simulink model "model_cnn"  (R2020a)
settings: Solver=VariableStepAuto  StartTime=0.0  StopTime=1e6/fs  RelTol=1e-3
PreLoadFcn:
  | setup_imports;
  | %dense2_numerictype = fixdt(1,18,10);
  | %conv1_numerictype = fixdt(1,18,21);
InitFcn:
  | % Intermediate signal dimensions
  | input_dim = [1, 2, 128];
  | layer1_dim = hInterConvLayerDims([1,3,1,64],input_dim,1); % dims : [C,H,W]
  | layer2_dim = hInterConvLayerDims([2,3,64,16],layer1_dim,1);% dims : [C,H,W]
  | layer3_dim = [1,128];
  | 
  | % Conv Layer 1 dimensions
  | conv1_dims = struct(...
  |     'input_dim',    input_dim,...       input_dim = C,H,W
  |     'filter_dim',   [1, 3, 1, 64],...  filter_dim = K,J,C,N
  |     'stride',       1,...
  |     'row_output',   3,...
  |     'output_dim',   layer1_dim);
  | 
  | % Conv Layer 2 dimensions
  | conv2_dims = struct(...
  |     'input_dim',    layer1_dim,...      input = C,H.W
  |     'filter_dim',   [2, 3, 64, 16],...  filter_dim = K,J,C,N
  |     'stride',       1,...
  |     'row_output',   2*3*64,...
  |     'output_dim',   layer2_dim);
  | 
  | % Dense Layer 1 dimensions
  | dense1_dims = struct(...
  |     'input_dim',    layer2_dim,...      input = C,H,W
  |     'weight_dim',   [1984, 128],...     weight_dim = H,W
  |     'output_dim',   layer3_dim);
  | 
  | % Load saved weights and input
  | setup_imports;
  | 
  | fs = 128e6;
  | fs_axi = 100e6;
  | R = 32;
values from neighbouring files (symbols this model uses):
  datatypeInput = X_test.numerictype    [setup_imports.m]
  gemm_wconv1 = fi(hInterleaveFilters(Wconv1),1,16)    [setup_imports.m]
  gemm_wconv2 = fi(hInterleaveFilters(Wconv2),1,16)    [setup_imports.m]
  wdense1 = fi(Wdense1,1,16)    [setup_imports.m]
  wdense2 = fi(Wdense2,1,16)    [setup_imports.m]
undefined symbols (not defined in the file or in its folder): ltehdlRAMinitPO2
libraries: hdlsllib x1022, dspsigops x3, dspsrcs4 x2
(part 9 of 23)

== system model_cnn/HDL CNN Model/Dense Layer 1/Dense Layer 1/Weight Storage79 ==
  count_Weights : Inport
  Constant : Constant  Value=0  OutDataTypeStr=wdense1.numerictype  SampleTime=-1
  Constant1 : Constant  Value=false  SampleTime=-1
  Single Port RAM System : hdlsllib/HDL RAMs/Single Port RAM System  RAMType=Single port  WriteOutputValue=New data  RAMInitialValue=ltehdlRAMinitPO2(wdense1(:,dim).',2048)  SimulateUsing=Code generation
      settings: SourceProductBaseCode=SL
  Out1 : Outport
  wires:
  Single Port RAM System/1 -> Out1/1
  Constant/1 -> Single Port RAM System/1
  Constant1/1 -> Single Port RAM System/3
  count_Weights/1 -> Single Port RAM System/2

== system model_cnn/HDL CNN Model/Dense Layer 1/Dense Layer 1/Weight Storage8 ==
  count_Weights : Inport
  Constant : Constant  Value=0  OutDataTypeStr=wdense1.numerictype  SampleTime=-1
  Constant1 : Constant  Value=false  SampleTime=-1
  Single Port RAM System : hdlsllib/HDL RAMs/Single Port RAM System  RAMType=Single port  WriteOutputValue=New data  RAMInitialValue=ltehdlRAMinitPO2(wdense1(:,dim).',2048)  SimulateUsing=Code generation
      settings: SourceProductBaseCode=SL
  Out1 : Outport
  wires:
  Single Port RAM System/1 -> Out1/1
  Constant/1 -> Single Port RAM System/1
  Constant1/1 -> Single Port RAM System/3
  count_Weights/1 -> Single Port RAM System/2

== system model_cnn/HDL CNN Model/Dense Layer 1/Dense Layer 1/Weight Storage80 ==
  count_Weights : Inport
  Constant : Constant  Value=0  OutDataTypeStr=wdense1.numerictype  SampleTime=-1
  Constant1 : Constant  Value=false  SampleTime=-1
  Single Port RAM System : hdlsllib/HDL RAMs/Single Port RAM System  RAMType=Single port  WriteOutputValue=New data  RAMInitialValue=ltehdlRAMinitPO2(wdense1(:,dim).',2048)  SimulateUsing=Code generation
      settings: SourceProductBaseCode=SL
  Out1 : Outport
  wires:
  Single Port RAM System/1 -> Out1/1
  Constant/1 -> Single Port RAM System/1
  Constant1/1 -> Single Port RAM System/3
  count_Weights/1 -> Single Port RAM System/2

== system model_cnn/HDL CNN Model/Dense Layer 1/Dense Layer 1/Weight Storage81 ==
  count_Weights : Inport
  Constant : Constant  Value=0  OutDataTypeStr=wdense1.numerictype  SampleTime=-1
  Constant1 : Constant  Value=false  SampleTime=-1
  Single Port RAM System : hdlsllib/HDL RAMs/Single Port RAM System  RAMType=Single port  WriteOutputValue=New data  RAMInitialValue=ltehdlRAMinitPO2(wdense1(:,dim).',2048)  SimulateUsing=Code generation
      settings: SourceProductBaseCode=SL
  Out1 : Outport
  wires:
  Single Port RAM System/1 -> Out1/1
  Constant/1 -> Single Port RAM System/1
  Constant1/1 -> Single Port RAM System/3
  count_Weights/1 -> Single Port RAM System/2

== system model_cnn/HDL CNN Model/Dense Layer 1/Dense Layer 1/Weight Storage82 ==
  count_Weights : Inport
  Constant : Constant  Value=0  OutDataTypeStr=wdense1.numerictype  SampleTime=-1
  Constant1 : Constant  Value=false  SampleTime=-1
  Single Port RAM System : hdlsllib/HDL RAMs/Single Port RAM System  RAMType=Single port  WriteOutputValue=New data  RAMInitialValue=ltehdlRAMinitPO2(wdense1(:,dim).',2048)  SimulateUsing=Code generation
      settings: SourceProductBaseCode=SL
  Out1 : Outport
  wires:
  Single Port RAM System/1 -> Out1/1
  Constant/1 -> Single Port RAM System/1
  Constant1/1 -> Single Port RAM System/3
  count_Weights/1 -> Single Port RAM System/2

== system model_cnn/HDL CNN Model/Dense Layer 1/Dense Layer 1/Weight Storage83 ==
  count_Weights : Inport
  Constant : Constant  Value=0  OutDataTypeStr=wdense1.numerictype  SampleTime=-1
  Constant1 : Constant  Value=false  SampleTime=-1
  Single Port RAM System : hdlsllib/HDL RAMs/Single Port RAM System  RAMType=Single port  WriteOutputValue=New data  RAMInitialValue=ltehdlRAMinitPO2(wdense1(:,dim).',2048)  SimulateUsing=Code generation
      settings: SourceProductBaseCode=SL
  Out1 : Outport
  wires:
  Single Port RAM System/1 -> Out1/1
  Constant/1 -> Single Port RAM System/1
  Constant1/1 -> Single Port RAM System/3
  count_Weights/1 -> Single Port RAM System/2

== system model_cnn/HDL CNN Model/Dense Layer 1/Dense Layer 1/Weight Storage84 ==
  count_Weights : Inport
  Constant : Constant  Value=0  OutDataTypeStr=wdense1.numerictype  SampleTime=-1
  Constant1 : Constant  Value=false  SampleTime=-1
  Single Port RAM System : hdlsllib/HDL RAMs/Single Port RAM System  RAMType=Single port  WriteOutputValue=New data  RAMInitialValue=ltehdlRAMinitPO2(wdense1(:,dim).',2048)  SimulateUsing=Code generation
      settings: SourceProductBaseCode=SL
  Out1 : Outport
  wires:
  Single Port RAM System/1 -> Out1/1
  Constant/1 -> Single Port RAM System/1
  Constant1/1 -> Single Port RAM System/3
  count_Weights/1 -> Single Port RAM System/2

== system model_cnn/HDL CNN Model/Dense Layer 1/Dense Layer 1/Weight Storage85 ==
  count_Weights : Inport
  Constant : Constant  Value=0  OutDataTypeStr=wdense1.numerictype  SampleTime=-1
  Constant1 : Constant  Value=false  SampleTime=-1
  Single Port RAM System : hdlsllib/HDL RAMs/Single Port RAM System  RAMType=Single port  WriteOutputValue=New data  RAMInitialValue=ltehdlRAMinitPO2(wdense1(:,dim).',2048)  SimulateUsing=Code generation
      settings: SourceProductBaseCode=SL
  Out1 : Outport
  wires:
  Single Port RAM System/1 -> Out1/1
  Constant/1 -> Single Port RAM System/1
  Constant1/1 -> Single Port RAM System/3
  count_Weights/1 -> Single Port RAM System/2

== system model_cnn/HDL CNN Model/Dense Layer 1/Dense Layer 1/Weight Storage86 ==
  count_Weights : Inport
  Constant : Constant  Value=0  OutDataTypeStr=wdense1.numerictype  SampleTime=-1
  Constant1 : Constant  Value=false  SampleTime=-1
  Single Port RAM System : hdlsllib/HDL RAMs/Single Port RAM System  RAMType=Single port  WriteOutputValue=New data  RAMInitialValue=ltehdlRAMinitPO2(wdense1(:,dim).',2048)  SimulateUsing=Code generation
      settings: SourceProductBaseCode=SL
  Out1 : Outport
  wires:
  Single Port RAM System/1 -> Out1/1
  Constant/1 -> Single Port RAM System/1
  Constant1/1 -> Single Port RAM System/3
  count_Weights/1 -> Single Port RAM System/2

== system model_cnn/HDL CNN Model/Dense Layer 1/Dense Layer 1/Weight Storage87 ==
  count_Weights : Inport
  Constant : Constant  Value=0  OutDataTypeStr=wdense1.numerictype  SampleTime=-1
  Constant1 : Constant  Value=false  SampleTime=-1
  Single Port RAM System : hdlsllib/HDL RAMs/Single Port RAM System  RAMType=Single port  WriteOutputValue=New data  RAMInitialValue=ltehdlRAMinitPO2(wdense1(:,dim).',2048)  SimulateUsing=Code generation
      settings: SourceProductBaseCode=SL
  Out1 : Outport
  wires:
  Single Port RAM System/1 -> Out1/1
  Constant/1 -> Single Port RAM System/1
  Constant1/1 -> Single Port RAM System/3
  count_Weights/1 -> Single Port RAM System/2

== system model_cnn/HDL CNN Model/Dense Layer 1/Dense Layer 1/Weight Storage88 ==
  count_Weights : Inport
  Constant : Constant  Value=0  OutDataTypeStr=wdense1.numerictype  SampleTime=-1
  Constant1 : Constant  Value=false  SampleTime=-1
  Single Port RAM System : hdlsllib/HDL RAMs/Single Port RAM System  RAMType=Single port  WriteOutputValue=New data  RAMInitialValue=ltehdlRAMinitPO2(wdense1(:,dim).',2048)  SimulateUsing=Code generation
      settings: SourceProductBaseCode=SL
  Out1 : Outport
  wires:
  Single Port RAM System/1 -> Out1/1
  Constant/1 -> Single Port RAM System/1
  Constant1/1 -> Single Port RAM System/3
  count_Weights/1 -> Single Port RAM System/2

== system model_cnn/HDL CNN Model/Dense Layer 1/Dense Layer 1/Weight Storage89 ==
  count_Weights : Inport
  Constant : Constant  Value=0  OutDataTypeStr=wdense1.numerictype  SampleTime=-1
  Constant1 : Constant  Value=false  SampleTime=-1
  Single Port RAM System : hdlsllib/HDL RAMs/Single Port RAM System  RAMType=Single port  WriteOutputValue=New data  RAMInitialValue=ltehdlRAMinitPO2(wdense1(:,dim).',2048)  SimulateUsing=Code generation
      settings: SourceProductBaseCode=SL
  Out1 : Outport
  wires:
  Single Port RAM System/1 -> Out1/1
  Constant/1 -> Single Port RAM System/1
  Constant1/1 -> Single Port RAM System/3
  count_Weights/1 -> Single Port RAM System/2

== system model_cnn/HDL CNN Model/Dense Layer 1/Dense Layer 1/Weight Storage9 ==
  count_Weights : Inport
  Constant : Constant  Value=0  OutDataTypeStr=wdense1.numerictype  SampleTime=-1
  Constant1 : Constant  Value=false  SampleTime=-1
  Single Port RAM System : hdlsllib/HDL RAMs/Single Port RAM System  RAMType=Single port  WriteOutputValue=New data  RAMInitialValue=ltehdlRAMinitPO2(wdense1(:,dim).',2048)  SimulateUsing=Code generation
      settings: SourceProductBaseCode=SL
  Out1 : Outport
  wires:
  Single Port RAM System/1 -> Out1/1
  Constant/1 -> Single Port RAM System/1
  Constant1/1 -> Single Port RAM System/3
  count_Weights/1 -> Single Port RAM System/2

== system model_cnn/HDL CNN Model/Dense Layer 1/Dense Layer 1/Weight Storage90 ==
  count_Weights : Inport
  Constant : Constant  Value=0  OutDataTypeStr=wdense1.numerictype  SampleTime=-1
  Constant1 : Constant  Value=false  SampleTime=-1
  Single Port RAM System : hdlsllib/HDL RAMs/Single Port RAM System  RAMType=Single port  WriteOutputValue=New data  RAMInitialValue=ltehdlRAMinitPO2(wdense1(:,dim).',2048)  SimulateUsing=Code generation
      settings: SourceProductBaseCode=SL
  Out1 : Outport
  wires:
  Single Port RAM System/1 -> Out1/1
  Constant/1 -> Single Port RAM System/1
  Constant1/1 -> Single Port RAM System/3
  count_Weights/1 -> Single Port RAM System/2

== system model_cnn/HDL CNN Model/Dense Layer 1/Dense Layer 1/Weight Storage91 ==
  count_Weights : Inport
  Constant : Constant  Value=0  OutDataTypeStr=wdense1.numerictype  SampleTime=-1
  Constant1 : Constant  Value=false  SampleTime=-1
  Single Port RAM System : hdlsllib/HDL RAMs/Single Port RAM System  RAMType=Single port  WriteOutputValue=New data  RAMInitialValue=ltehdlRAMinitPO2(wdense1(:,dim).',2048)  SimulateUsing=Code generation
      settings: SourceProductBaseCode=SL
  Out1 : Outport
  wires:
  Single Port RAM System/1 -> Out1/1
  Constant/1 -> Single Port RAM System/1
  Constant1/1 -> Single Port RAM System/3
  count_Weights/1 -> Single Port RAM System/2

== system model_cnn/HDL CNN Model/Dense Layer 1/Dense Layer 1/Weight Storage92 ==
  count_Weights : Inport
  Constant : Constant  Value=0  OutDataTypeStr=wdense1.numerictype  SampleTime=-1
  Constant1 : Constant  Value=false  SampleTime=-1
  Single Port RAM System : hdlsllib/HDL RAMs/Single Port RAM System  RAMType=Single port  WriteOutputValue=New data  RAMInitialValue=ltehdlRAMinitPO2(wdense1(:,dim).',2048)  SimulateUsing=Code generation
      settings: SourceProductBaseCode=SL
  Out1 : Outport
  wires:
  Single Port RAM System/1 -> Out1/1
  Constant/1 -> Single Port RAM System/1
  Constant1/1 -> Single Port RAM System/3
  count_Weights/1 -> Single Port RAM System/2

== system model_cnn/HDL CNN Model/Dense Layer 1/Dense Layer 1/Weight Storage93 ==
  count_Weights : Inport
  Constant : Constant  Value=0  OutDataTypeStr=wdense1.numerictype  SampleTime=-1
  Constant1 : Constant  Value=false  SampleTime=-1
  Single Port RAM System : hdlsllib/HDL RAMs/Single Port RAM System  RAMType=Single port  WriteOutputValue=New data  RAMInitialValue=ltehdlRAMinitPO2(wdense1(:,dim).',2048)  SimulateUsing=Code generation
      settings: SourceProductBaseCode=SL
  Out1 : Outport
  wires:
  Single Port RAM System/1 -> Out1/1
  Constant/1 -> Single Port RAM System/1
  Constant1/1 -> Single Port RAM System/3
  count_Weights/1 -> Single Port RAM System/2

== system model_cnn/HDL CNN Model/Dense Layer 1/Dense Layer 1/Weight Storage94 ==
  count_Weights : Inport
  Constant : Constant  Value=0  OutDataTypeStr=wdense1.numerictype  SampleTime=-1
  Constant1 : Constant  Value=false  SampleTime=-1
  Single Port RAM System : hdlsllib/HDL RAMs/Single Port RAM System  RAMType=Single port  WriteOutputValue=New data  RAMInitialValue=ltehdlRAMinitPO2(wdense1(:,dim).',2048)  SimulateUsing=Code generation
      settings: SourceProductBaseCode=SL
  Out1 : Outport
  wires:
  Single Port RAM System/1 -> Out1/1
  Constant/1 -> Single Port RAM System/1
  Constant1/1 -> Single Port RAM System/3
  count_Weights/1 -> Single Port RAM System/2

== system model_cnn/HDL CNN Model/Dense Layer 1/Dense Layer 1/Weight Storage95 ==
  count_Weights : Inport
  Constant : Constant  Value=0  OutDataTypeStr=wdense1.numerictype  SampleTime=-1
  Constant1 : Constant  Value=false  SampleTime=-1
  Single Port RAM System : hdlsllib/HDL RAMs/Single Port RAM System  RAMType=Single port  WriteOutputValue=New data  RAMInitialValue=ltehdlRAMinitPO2(wdense1(:,dim).',2048)  SimulateUsing=Code generation
      settings: SourceProductBaseCode=SL
  Out1 : Outport
  wires:
  Single Port RAM System/1 -> Out1/1
  Constant/1 -> Single Port RAM System/1
  Constant1/1 -> Single Port RAM System/3
  count_Weights/1 -> Single Port RAM System/2

== system model_cnn/HDL CNN Model/Dense Layer 1/Dense Layer 1/Weight Storage96 ==
  count_Weights : Inport
  Constant : Constant  Value=0  OutDataTypeStr=wdense1.numerictype  SampleTime=-1
  Constant1 : Constant  Value=false  SampleTime=-1
  Single Port RAM System : hdlsllib/HDL RAMs/Single Port RAM System  RAMType=Single port  WriteOutputValue=New data  RAMInitialValue=ltehdlRAMinitPO2(wdense1(:,dim).',2048)  SimulateUsing=Code generation
      settings: SourceProductBaseCode=SL
  Out1 : Outport
  wires:
  Single Port RAM System/1 -> Out1/1
  Constant/1 -> Single Port RAM System/1
  Constant1/1 -> Single Port RAM System/3
  count_Weights/1 -> Single Port RAM System/2

== system model_cnn/HDL CNN Model/Dense Layer 1/Dense Layer 1/Weight Storage97 ==
  count_Weights : Inport
  Constant : Constant  Value=0  OutDataTypeStr=wdense1.numerictype  SampleTime=-1
  Constant1 : Constant  Value=false  SampleTime=-1
  Single Port RAM System : hdlsllib/HDL RAMs/Single Port RAM System  RAMType=Single port  WriteOutputValue=New data  RAMInitialValue=ltehdlRAMinitPO2(wdense1(:,dim).',2048)  SimulateUsing=Code generation
      settings: SourceProductBaseCode=SL
  Out1 : Outport
  wires:
  Single Port RAM System/1 -> Out1/1
  Constant/1 -> Single Port RAM System/1
  Constant1/1 -> Single Port RAM System/3
  count_Weights/1 -> Single Port RAM System/2

== system model_cnn/HDL CNN Model/Dense Layer 1/Dense Layer 1/Weight Storage98 ==
  count_Weights : Inport
  Constant : Constant  Value=0  OutDataTypeStr=wdense1.numerictype  SampleTime=-1
  Constant1 : Constant  Value=false  SampleTime=-1
  Single Port RAM System : hdlsllib/HDL RAMs/Single Port RAM System  RAMType=Single port  WriteOutputValue=New data  RAMInitialValue=ltehdlRAMinitPO2(wdense1(:,dim).',2048)  SimulateUsing=Code generation
      settings: SourceProductBaseCode=SL
  Out1 : Outport
  wires:
  Single Port RAM System/1 -> Out1/1
  Constant/1 -> Single Port RAM System/1
  Constant1/1 -> Single Port RAM System/3
  count_Weights/1 -> Single Port RAM System/2

== system model_cnn/HDL CNN Model/Dense Layer 1/Dense Layer 1/Weight Storage99 ==
  count_Weights : Inport
  Constant : Constant  Value=0  OutDataTypeStr=wdense1.numerictype  SampleTime=-1
  Constant1 : Constant  Value=false  SampleTime=-1
  Single Port RAM System : hdlsllib/HDL RAMs/Single Port RAM System  RAMType=Single port  WriteOutputValue=New data  RAMInitialValue=ltehdlRAMinitPO2(wdense1(:,dim).',2048)  SimulateUsing=Code generation
      settings: SourceProductBaseCode=SL
  Out1 : Outport
  wires:
  Single Port RAM System/1 -> Out1/1
  Constant/1 -> Single Port RAM System/1
  Constant1/1 -> Single Port RAM System/3
  count_Weights/1 -> Single Port RAM System/2

== system model_cnn/HDL CNN Model/Dense Layer 1/Dense Layer 1/adder 0 ==
  In1 : Inport
  In2 : Inport  Port=2
  In3 : Inport  Port=3
  Data Type Conversion : DataTypeConversion  OutDataTypeStr=datatypeLayer3
  Multiply-Accumulate : hdlsllib/HDL Operations/Multiply-Accumulate  opMode=Streaming - using Number of Samples  initValueSetting=Dialog  initValue=0  initValueSetting2=Dialog  initValue2=0  initValueSetting3=Dialog  initValue3=0  num_samples=1984  RndMeth2=Floor  RndMeth3=Floor  datatype2=Inherit: Inherit via back propagation  datatype3=accumoutdatatype3  validOut=on  endInandOut=on  startOut=on  countOut=on  dim=-1  DoSatur=off  parallel=off
      settings: SourceProductBaseCode=SL
  Terminator : Terminator
  Terminator1 : Terminator
  dataOut : Outport
  validOut : Outport  Port=2
  wires:
  ? -> validOut/1  "vectorOutValid"
  In1/1 -> Multiply-Accumulate/2
  ? -> Terminator/1  "countOut"
  Multiply-Accumulate/1 -> Data Type Conversion/1
  In3/1 -> ?
  In2/1 -> Multiply-Accumulate/1
  ? -> Terminator1/1  "validOut"
  Data Type Conversion/1 -> dataOut/1

== system model_cnn/HDL CNN Model/Dense Layer 1/Dense Layer 1/adder1 ==
  In1 : Inport
  In2 : Inport  Port=2
  In3 : Inport  Port=3
  Data Type Conversion : DataTypeConversion  OutDataTypeStr=datatypeLayer3
  Multiply-Accumulate : hdlsllib/HDL Operations/Multiply-Accumulate  opMode=Streaming - using Number of Samples  initValueSetting=Dialog  initValue=0  initValueSetting2=Dialog  initValue2=0  initValueSetting3=Dialog  initValue3=0  num_samples=1984  RndMeth2=Floor  RndMeth3=Floor  datatype2=Inherit: Inherit via back propagation  datatype3=accumoutdatatype3  validOut=on  endInandOut=on  startOut=on  countOut=on  dim=-1  DoSatur=off  parallel=off
      settings: SourceProductBaseCode=SL
  Terminator : Terminator
  Terminator1 : Terminator
  Terminator2 : Terminator
  dataOut : Outport
  wires:
  Data Type Conversion/1 -> dataOut/1
  ? -> Terminator1/1  "validOut"
  In2/1 -> Multiply-Accumulate/1
  In3/1 -> ?
  Multiply-Accumulate/1 -> Data Type Conversion/1
  ? -> Terminator/1  "countOut"
  In1/1 -> Multiply-Accumulate/2
  ? -> Terminator2/1  "vectorOutValid"

== system model_cnn/HDL CNN Model/Dense Layer 1/Dense Layer 1/adder10 ==
  In1 : Inport
  In2 : Inport  Port=2
  In3 : Inport  Port=3
  Data Type Conversion : DataTypeConversion  OutDataTypeStr=datatypeLayer3
  Multiply-Accumulate : hdlsllib/HDL Operations/Multiply-Accumulate  opMode=Streaming - using Number of Samples  initValueSetting=Dialog  initValue=0  initValueSetting2=Dialog  initValue2=0  initValueSetting3=Dialog  initValue3=0  num_samples=1984  RndMeth2=Floor  RndMeth3=Floor  datatype2=Inherit: Inherit via back propagation  datatype3=accumoutdatatype3  validOut=on  endInandOut=on  startOut=on  countOut=on  dim=-1  DoSatur=off  parallel=off
      settings: SourceProductBaseCode=SL
  Terminator : Terminator
  Terminator1 : Terminator
  Terminator2 : Terminator
  dataOut : Outport
  wires:
  Data Type Conversion/1 -> dataOut/1
  ? -> Terminator1/1  "validOut"
  In2/1 -> Multiply-Accumulate/1
  In3/1 -> ?
  Multiply-Accumulate/1 -> Data Type Conversion/1
  ? -> Terminator/1  "countOut"
  In1/1 -> Multiply-Accumulate/2
  ? -> Terminator2/1  "vectorOutValid"

== system model_cnn/HDL CNN Model/Dense Layer 1/Dense Layer 1/adder100 ==
  In1 : Inport
  In2 : Inport  Port=2
  In3 : Inport  Port=3
  Data Type Conversion : DataTypeConversion  OutDataTypeStr=datatypeLayer3
  Multiply-Accumulate : hdlsllib/HDL Operations/Multiply-Accumulate  opMode=Streaming - using Number of Samples  initValueSetting=Dialog  initValue=0  initValueSetting2=Dialog  initValue2=0  initValueSetting3=Dialog  initValue3=0  num_samples=1984  RndMeth2=Floor  RndMeth3=Floor  datatype2=Inherit: Inherit via back propagation  datatype3=accumoutdatatype3  validOut=on  endInandOut=on  startOut=on  countOut=on  dim=-1  DoSatur=off  parallel=off
      settings: SourceProductBaseCode=SL
  Terminator : Terminator
  Terminator1 : Terminator
  Terminator2 : Terminator
  dataOut : Outport
  wires:
  Data Type Conversion/1 -> dataOut/1
  ? -> Terminator1/1  "validOut"
  In2/1 -> Multiply-Accumulate/1
  In3/1 -> ?
  Multiply-Accumulate/1 -> Data Type Conversion/1
  ? -> Terminator/1  "countOut"
  In1/1 -> Multiply-Accumulate/2
  ? -> Terminator2/1  "vectorOutValid"

== system model_cnn/HDL CNN Model/Dense Layer 1/Dense Layer 1/adder101 ==
  In1 : Inport
  In2 : Inport  Port=2
  In3 : Inport  Port=3
  Data Type Conversion : DataTypeConversion  OutDataTypeStr=datatypeLayer3
  Multiply-Accumulate : hdlsllib/HDL Operations/Multiply-Accumulate  opMode=Streaming - using Number of Samples  initValueSetting=Dialog  initValue=0  initValueSetting2=Dialog  initValue2=0  initValueSetting3=Dialog  initValue3=0  num_samples=1984  RndMeth2=Floor  RndMeth3=Floor  datatype2=Inherit: Inherit via back propagation  datatype3=accumoutdatatype3  validOut=on  endInandOut=on  startOut=on  countOut=on  dim=-1  DoSatur=off  parallel=off
      settings: SourceProductBaseCode=SL
  Terminator : Terminator
  Terminator1 : Terminator
  Terminator2 : Terminator
  dataOut : Outport
  wires:
  Data Type Conversion/1 -> dataOut/1
  ? -> Terminator1/1  "validOut"
  In2/1 -> Multiply-Accumulate/1
  In3/1 -> ?
  Multiply-Accumulate/1 -> Data Type Conversion/1
  ? -> Terminator/1  "countOut"
  In1/1 -> Multiply-Accumulate/2
  ? -> Terminator2/1  "vectorOutValid"

== system model_cnn/HDL CNN Model/Dense Layer 1/Dense Layer 1/adder102 ==
  In1 : Inport
  In2 : Inport  Port=2
  In3 : Inport  Port=3
  Data Type Conversion : DataTypeConversion  OutDataTypeStr=datatypeLayer3
  Multiply-Accumulate : hdlsllib/HDL Operations/Multiply-Accumulate  opMode=Streaming - using Number of Samples  initValueSetting=Dialog  initValue=0  initValueSetting2=Dialog  initValue2=0  initValueSetting3=Dialog  initValue3=0  num_samples=1984  RndMeth2=Floor  RndMeth3=Floor  datatype2=Inherit: Inherit via back propagation  datatype3=accumoutdatatype3  validOut=on  endInandOut=on  startOut=on  countOut=on  dim=-1  DoSatur=off  parallel=off
      settings: SourceProductBaseCode=SL
  Terminator : Terminator
  Terminator1 : Terminator
  Terminator2 : Terminator
  dataOut : Outport
  wires:
  Data Type Conversion/1 -> dataOut/1
  ? -> Terminator1/1  "validOut"
  In2/1 -> Multiply-Accumulate/1
  In3/1 -> ?
  Multiply-Accumulate/1 -> Data Type Conversion/1
  ? -> Terminator/1  "countOut"
  In1/1 -> Multiply-Accumulate/2
  ? -> Terminator2/1  "vectorOutValid"

== system model_cnn/HDL CNN Model/Dense Layer 1/Dense Layer 1/adder103 ==
  In1 : Inport
  In2 : Inport  Port=2
  In3 : Inport  Port=3
  Data Type Conversion : DataTypeConversion  OutDataTypeStr=datatypeLayer3
  Multiply-Accumulate : hdlsllib/HDL Operations/Multiply-Accumulate  opMode=Streaming - using Number of Samples  initValueSetting=Dialog  initValue=0  initValueSetting2=Dialog  initValue2=0  initValueSetting3=Dialog  initValue3=0  num_samples=1984  RndMeth2=Floor  RndMeth3=Floor  datatype2=Inherit: Inherit via back propagation  datatype3=accumoutdatatype3  validOut=on  endInandOut=on  startOut=on  countOut=on  dim=-1  DoSatur=off  parallel=off
      settings: SourceProductBaseCode=SL
  Terminator : Terminator
  Terminator1 : Terminator
  Terminator2 : Terminator
  dataOut : Outport
  wires:
  Data Type Conversion/1 -> dataOut/1
  ? -> Terminator1/1  "validOut"
  In2/1 -> Multiply-Accumulate/1
  In3/1 -> ?
  Multiply-Accumulate/1 -> Data Type Conversion/1
  ? -> Terminator/1  "countOut"
  In1/1 -> Multiply-Accumulate/2
  ? -> Terminator2/1  "vectorOutValid"

== system model_cnn/HDL CNN Model/Dense Layer 1/Dense Layer 1/adder104 ==
  In1 : Inport
  In2 : Inport  Port=2
  In3 : Inport  Port=3
  Data Type Conversion : DataTypeConversion  OutDataTypeStr=datatypeLayer3
  Multiply-Accumulate : hdlsllib/HDL Operations/Multiply-Accumulate  opMode=Streaming - using Number of Samples  initValueSetting=Dialog  initValue=0  initValueSetting2=Dialog  initValue2=0  initValueSetting3=Dialog  initValue3=0  num_samples=1984  RndMeth2=Floor  RndMeth3=Floor  datatype2=Inherit: Inherit via back propagation  datatype3=accumoutdatatype3  validOut=on  endInandOut=on  startOut=on  countOut=on  dim=-1  DoSatur=off  parallel=off
      settings: SourceProductBaseCode=SL
  Terminator : Terminator
  Terminator1 : Terminator
  Terminator2 : Terminator
  dataOut : Outport
  wires:
  Data Type Conversion/1 -> dataOut/1
  ? -> Terminator1/1  "validOut"
  In2/1 -> Multiply-Accumulate/1
  In3/1 -> ?
  Multiply-Accumulate/1 -> Data Type Conversion/1
  ? -> Terminator/1  "countOut"
  In1/1 -> Multiply-Accumulate/2
  ? -> Terminator2/1  "vectorOutValid"

== system model_cnn/HDL CNN Model/Dense Layer 1/Dense Layer 1/adder105 ==
  In1 : Inport
  In2 : Inport  Port=2
  In3 : Inport  Port=3
  Data Type Conversion : DataTypeConversion  OutDataTypeStr=datatypeLayer3
  Multiply-Accumulate : hdlsllib/HDL Operations/Multiply-Accumulate  opMode=Streaming - using Number of Samples  initValueSetting=Dialog  initValue=0  initValueSetting2=Dialog  initValue2=0  initValueSetting3=Dialog  initValue3=0  num_samples=1984  RndMeth2=Floor  RndMeth3=Floor  datatype2=Inherit: Inherit via back propagation  datatype3=accumoutdatatype3  validOut=on  endInandOut=on  startOut=on  countOut=on  dim=-1  DoSatur=off  parallel=off
      settings: SourceProductBaseCode=SL
  Terminator : Terminator
  Terminator1 : Terminator
  Terminator2 : Terminator
  dataOut : Outport
  wires:
  Data Type Conversion/1 -> dataOut/1
  ? -> Terminator1/1  "validOut"
  In2/1 -> Multiply-Accumulate/1
  In3/1 -> ?
  Multiply-Accumulate/1 -> Data Type Conversion/1
  ? -> Terminator/1  "countOut"
  In1/1 -> Multiply-Accumulate/2
  ? -> Terminator2/1  "vectorOutValid"

== system model_cnn/HDL CNN Model/Dense Layer 1/Dense Layer 1/adder106 ==
  In1 : Inport
  In2 : Inport  Port=2
  In3 : Inport  Port=3
  Data Type Conversion : DataTypeConversion  OutDataTypeStr=datatypeLayer3
  Multiply-Accumulate : hdlsllib/HDL Operations/Multiply-Accumulate  opMode=Streaming - using Number of Samples  initValueSetting=Dialog  initValue=0  initValueSetting2=Dialog  initValue2=0  initValueSetting3=Dialog  initValue3=0  num_samples=1984  RndMeth2=Floor  RndMeth3=Floor  datatype2=Inherit: Inherit via back propagation  datatype3=accumoutdatatype3  validOut=on  endInandOut=on  startOut=on  countOut=on  dim=-1  DoSatur=off  parallel=off
      settings: SourceProductBaseCode=SL
  Terminator : Terminator
  Terminator1 : Terminator
  Terminator2 : Terminator
  dataOut : Outport
  wires:
  Data Type Conversion/1 -> dataOut/1
  ? -> Terminator1/1  "validOut"
  In2/1 -> Multiply-Accumulate/1
  In3/1 -> ?
  Multiply-Accumulate/1 -> Data Type Conversion/1
  ? -> Terminator/1  "countOut"
  In1/1 -> Multiply-Accumulate/2
  ? -> Terminator2/1  "vectorOutValid"

== system model_cnn/HDL CNN Model/Dense Layer 1/Dense Layer 1/adder107 ==
  In1 : Inport
  In2 : Inport  Port=2
  In3 : Inport  Port=3
  Data Type Conversion : DataTypeConversion  OutDataTypeStr=datatypeLayer3
  Multiply-Accumulate : hdlsllib/HDL Operations/Multiply-Accumulate  opMode=Streaming - using Number of Samples  initValueSetting=Dialog  initValue=0  initValueSetting2=Dialog  initValue2=0  initValueSetting3=Dialog  initValue3=0  num_samples=1984  RndMeth2=Floor  RndMeth3=Floor  datatype2=Inherit: Inherit via back propagation  datatype3=accumoutdatatype3  validOut=on  endInandOut=on  startOut=on  countOut=on  dim=-1  DoSatur=off  parallel=off
      settings: SourceProductBaseCode=SL
  Terminator : Terminator
  Terminator1 : Terminator
  Terminator2 : Terminator
  dataOut : Outport
  wires:
  Data Type Conversion/1 -> dataOut/1
  ? -> Terminator1/1  "validOut"
  In2/1 -> Multiply-Accumulate/1
  In3/1 -> ?
  Multiply-Accumulate/1 -> Data Type Conversion/1
  ? -> Terminator/1  "countOut"
  In1/1 -> Multiply-Accumulate/2
  ? -> Terminator2/1  "vectorOutValid"

== system model_cnn/HDL CNN Model/Dense Layer 1/Dense Layer 1/adder108 ==
  In1 : Inport
  In2 : Inport  Port=2
  In3 : Inport  Port=3
  Data Type Conversion : DataTypeConversion  OutDataTypeStr=datatypeLayer3
  Multiply-Accumulate : hdlsllib/HDL Operations/Multiply-Accumulate  opMode=Streaming - using Number of Samples  initValueSetting=Dialog  initValue=0  initValueSetting2=Dialog  initValue2=0  initValueSetting3=Dialog  initValue3=0  num_samples=1984  RndMeth2=Floor  RndMeth3=Floor  datatype2=Inherit: Inherit via back propagation  datatype3=accumoutdatatype3  validOut=on  endInandOut=on  startOut=on  countOut=on  dim=-1  DoSatur=off  parallel=off
      settings: SourceProductBaseCode=SL
  Terminator : Terminator
  Terminator1 : Terminator
  Terminator2 : Terminator
  dataOut : Outport
  wires:
  Data Type Conversion/1 -> dataOut/1
  ? -> Terminator1/1  "validOut"
  In2/1 -> Multiply-Accumulate/1
  In3/1 -> ?
  Multiply-Accumulate/1 -> Data Type Conversion/1
  ? -> Terminator/1  "countOut"
  In1/1 -> Multiply-Accumulate/2
  ? -> Terminator2/1  "vectorOutValid"

== system model_cnn/HDL CNN Model/Dense Layer 1/Dense Layer 1/adder109 ==
  In1 : Inport
  In2 : Inport  Port=2
  In3 : Inport  Port=3
  Data Type Conversion : DataTypeConversion  OutDataTypeStr=datatypeLayer3
  Multiply-Accumulate : hdlsllib/HDL Operations/Multiply-Accumulate  opMode=Streaming - using Number of Samples  initValueSetting=Dialog  initValue=0  initValueSetting2=Dialog  initValue2=0  initValueSetting3=Dialog  initValue3=0  num_samples=1984  RndMeth2=Floor  RndMeth3=Floor  datatype2=Inherit: Inherit via back propagation  datatype3=accumoutdatatype3  validOut=on  endInandOut=on  startOut=on  countOut=on  dim=-1  DoSatur=off  parallel=off
      settings: SourceProductBaseCode=SL
  Terminator : Terminator
  Terminator1 : Terminator
  Terminator2 : Terminator
  dataOut : Outport
  wires:
  Data Type Conversion/1 -> dataOut/1
  ? -> Terminator1/1  "validOut"
  In2/1 -> Multiply-Accumulate/1
  In3/1 -> ?
  Multiply-Accumulate/1 -> Data Type Conversion/1
  ? -> Terminator/1  "countOut"
  In1/1 -> Multiply-Accumulate/2
  ? -> Terminator2/1  "vectorOutValid"

== system model_cnn/HDL CNN Model/Dense Layer 1/Dense Layer 1/adder11 ==
  In1 : Inport
  In2 : Inport  Port=2
  In3 : Inport  Port=3
  Data Type Conversion : DataTypeConversion  OutDataTypeStr=datatypeLayer3
  Multiply-Accumulate : hdlsllib/HDL Operations/Multiply-Accumulate  opMode=Streaming - using Number of Samples  initValueSetting=Dialog  initValue=0  initValueSetting2=Dialog  initValue2=0  initValueSetting3=Dialog  initValue3=0  num_samples=1984  RndMeth2=Floor  RndMeth3=Floor  datatype2=Inherit: Inherit via back propagation  datatype3=accumoutdatatype3  validOut=on  endInandOut=on  startOut=on  countOut=on  dim=-1  DoSatur=off  parallel=off
      settings: SourceProductBaseCode=SL
  Terminator : Terminator
  Terminator1 : Terminator
  Terminator2 : Terminator
  dataOut : Outport
  wires:
  Data Type Conversion/1 -> dataOut/1
  ? -> Terminator1/1  "validOut"
  In2/1 -> Multiply-Accumulate/1
  In3/1 -> ?
  Multiply-Accumulate/1 -> Data Type Conversion/1
  ? -> Terminator/1  "countOut"
  In1/1 -> Multiply-Accumulate/2
  ? -> Terminator2/1  "vectorOutValid"

== system model_cnn/HDL CNN Model/Dense Layer 1/Dense Layer 1/adder110 ==
  In1 : Inport
  In2 : Inport  Port=2
  In3 : Inport  Port=3
  Data Type Conversion : DataTypeConversion  OutDataTypeStr=datatypeLayer3
  Multiply-Accumulate : hdlsllib/HDL Operations/Multiply-Accumulate  opMode=Streaming - using Number of Samples  initValueSetting=Dialog  initValue=0  initValueSetting2=Dialog  initValue2=0  initValueSetting3=Dialog  initValue3=0  num_samples=1984  RndMeth2=Floor  RndMeth3=Floor  datatype2=Inherit: Inherit via back propagation  datatype3=accumoutdatatype3  validOut=on  endInandOut=on  startOut=on  countOut=on  dim=-1  DoSatur=off  parallel=off
      settings: SourceProductBaseCode=SL
  Terminator : Terminator
  Terminator1 : Terminator
  Terminator2 : Terminator
  dataOut : Outport
  wires:
  Data Type Conversion/1 -> dataOut/1
  ? -> Terminator1/1  "validOut"
  In2/1 -> Multiply-Accumulate/1
  In3/1 -> ?
  Multiply-Accumulate/1 -> Data Type Conversion/1
  ? -> Terminator/1  "countOut"
  In1/1 -> Multiply-Accumulate/2
  ? -> Terminator2/1  "vectorOutValid"

== system model_cnn/HDL CNN Model/Dense Layer 1/Dense Layer 1/adder111 ==
  In1 : Inport
  In2 : Inport  Port=2
  In3 : Inport  Port=3
  Data Type Conversion : DataTypeConversion  OutDataTypeStr=datatypeLayer3
  Multiply-Accumulate : hdlsllib/HDL Operations/Multiply-Accumulate  opMode=Streaming - using Number of Samples  initValueSetting=Dialog  initValue=0  initValueSetting2=Dialog  initValue2=0  initValueSetting3=Dialog  initValue3=0  num_samples=1984  RndMeth2=Floor  RndMeth3=Floor  datatype2=Inherit: Inherit via back propagation  datatype3=accumoutdatatype3  validOut=on  endInandOut=on  startOut=on  countOut=on  dim=-1  DoSatur=off  parallel=off
      settings: SourceProductBaseCode=SL
  Terminator : Terminator
  Terminator1 : Terminator
  Terminator2 : Terminator
  dataOut : Outport
  wires:
  Data Type Conversion/1 -> dataOut/1
  ? -> Terminator1/1  "validOut"
  In2/1 -> Multiply-Accumulate/1
  In3/1 -> ?
  Multiply-Accumulate/1 -> Data Type Conversion/1
  ? -> Terminator/1  "countOut"
  In1/1 -> Multiply-Accumulate/2
  ? -> Terminator2/1  "vectorOutValid"

== system model_cnn/HDL CNN Model/Dense Layer 1/Dense Layer 1/adder112 ==
  In1 : Inport
  In2 : Inport  Port=2
  In3 : Inport  Port=3
  Data Type Conversion : DataTypeConversion  OutDataTypeStr=datatypeLayer3
  Multiply-Accumulate : hdlsllib/HDL Operations/Multiply-Accumulate  opMode=Streaming - using Number of Samples  initValueSetting=Dialog  initValue=0  initValueSetting2=Dialog  initValue2=0  initValueSetting3=Dialog  initValue3=0  num_samples=1984  RndMeth2=Floor  RndMeth3=Floor  datatype2=Inherit: Inherit via back propagation  datatype3=accumoutdatatype3  validOut=on  endInandOut=on  startOut=on  countOut=on  dim=-1  DoSatur=off  parallel=off
      settings: SourceProductBaseCode=SL
  Terminator : Terminator
  Terminator1 : Terminator
  Terminator2 : Terminator
  dataOut : Outport
  wires:
  Data Type Conversion/1 -> dataOut/1
  ? -> Terminator1/1  "validOut"
  In2/1 -> Multiply-Accumulate/1
  In3/1 -> ?
  Multiply-Accumulate/1 -> Data Type Conversion/1
  ? -> Terminator/1  "countOut"
  In1/1 -> Multiply-Accumulate/2
  ? -> Terminator2/1  "vectorOutValid"

== system model_cnn/HDL CNN Model/Dense Layer 1/Dense Layer 1/adder113 ==
  In1 : Inport
  In2 : Inport  Port=2
  In3 : Inport  Port=3
  Data Type Conversion : DataTypeConversion  OutDataTypeStr=datatypeLayer3
  Multiply-Accumulate : hdlsllib/HDL Operations/Multiply-Accumulate  opMode=Streaming - using Number of Samples  initValueSetting=Dialog  initValue=0  initValueSetting2=Dialog  initValue2=0  initValueSetting3=Dialog  initValue3=0  num_samples=1984  RndMeth2=Floor  RndMeth3=Floor  datatype2=Inherit: Inherit via back propagation  datatype3=accumoutdatatype3  validOut=on  endInandOut=on  startOut=on  countOut=on  dim=-1  DoSatur=off  parallel=off
      settings: SourceProductBaseCode=SL
  Terminator : Terminator
  Terminator1 : Terminator
  Terminator2 : Terminator
  dataOut : Outport
  wires:
  Data Type Conversion/1 -> dataOut/1
  ? -> Terminator1/1  "validOut"
  In2/1 -> Multiply-Accumulate/1
  In3/1 -> ?
  Multiply-Accumulate/1 -> Data Type Conversion/1
  ? -> Terminator/1  "countOut"
  In1/1 -> Multiply-Accumulate/2
  ? -> Terminator2/1  "vectorOutValid"

== system model_cnn/HDL CNN Model/Dense Layer 1/Dense Layer 1/adder114 ==
  In1 : Inport
  In2 : Inport  Port=2
  In3 : Inport  Port=3
  Data Type Conversion : DataTypeConversion  OutDataTypeStr=datatypeLayer3
  Multiply-Accumulate : hdlsllib/HDL Operations/Multiply-Accumulate  opMode=Streaming - using Number of Samples  initValueSetting=Dialog  initValue=0  initValueSetting2=Dialog  initValue2=0  initValueSetting3=Dialog  initValue3=0  num_samples=1984  RndMeth2=Floor  RndMeth3=Floor  datatype2=Inherit: Inherit via back propagation  datatype3=accumoutdatatype3  validOut=on  endInandOut=on  startOut=on  countOut=on  dim=-1  DoSatur=off  parallel=off
      settings: SourceProductBaseCode=SL
  Terminator : Terminator
  Terminator1 : Terminator
  Terminator2 : Terminator
  dataOut : Outport
  wires:
  Data Type Conversion/1 -> dataOut/1
  ? -> Terminator1/1  "validOut"
  In2/1 -> Multiply-Accumulate/1
  In3/1 -> ?
  Multiply-Accumulate/1 -> Data Type Conversion/1
  ? -> Terminator/1  "countOut"
  In1/1 -> Multiply-Accumulate/2
  ? -> Terminator2/1  "vectorOutValid"

== system model_cnn/HDL CNN Model/Dense Layer 1/Dense Layer 1/adder115 ==
  In1 : Inport
  In2 : Inport  Port=2
  In3 : Inport  Port=3
  Data Type Conversion : DataTypeConversion  OutDataTypeStr=datatypeLayer3
  Multiply-Accumulate : hdlsllib/HDL Operations/Multiply-Accumulate  opMode=Streaming - using Number of Samples  initValueSetting=Dialog  initValue=0  initValueSetting2=Dialog  initValue2=0  initValueSetting3=Dialog  initValue3=0  num_samples=1984  RndMeth2=Floor  RndMeth3=Floor  datatype2=Inherit: Inherit via back propagation  datatype3=accumoutdatatype3  validOut=on  endInandOut=on  startOut=on  countOut=on  dim=-1  DoSatur=off  parallel=off
      settings: SourceProductBaseCode=SL
  Terminator : Terminator
  Terminator1 : Terminator
  Terminator2 : Terminator
  dataOut : Outport
  wires:
  Data Type Conversion/1 -> dataOut/1
  ? -> Terminator1/1  "validOut"
  In2/1 -> Multiply-Accumulate/1
  In3/1 -> ?
  Multiply-Accumulate/1 -> Data Type Conversion/1
  ? -> Terminator/1  "countOut"
  In1/1 -> Multiply-Accumulate/2
  ? -> Terminator2/1  "vectorOutValid"

== system model_cnn/HDL CNN Model/Dense Layer 1/Dense Layer 1/adder116 ==
  In1 : Inport
  In2 : Inport  Port=2
  In3 : Inport  Port=3
  Data Type Conversion : DataTypeConversion  OutDataTypeStr=datatypeLayer3
  Multiply-Accumulate : hdlsllib/HDL Operations/Multiply-Accumulate  opMode=Streaming - using Number of Samples  initValueSetting=Dialog  initValue=0  initValueSetting2=Dialog  initValue2=0  initValueSetting3=Dialog  initValue3=0  num_samples=1984  RndMeth2=Floor  RndMeth3=Floor  datatype2=Inherit: Inherit via back propagation  datatype3=accumoutdatatype3  validOut=on  endInandOut=on  startOut=on  countOut=on  dim=-1  DoSatur=off  parallel=off
      settings: SourceProductBaseCode=SL
  Terminator : Terminator
  Terminator1 : Terminator
  Terminator2 : Terminator
  dataOut : Outport
  wires:
  Data Type Conversion/1 -> dataOut/1
  ? -> Terminator1/1  "validOut"
  In2/1 -> Multiply-Accumulate/1
  In3/1 -> ?
  Multiply-Accumulate/1 -> Data Type Conversion/1
  ? -> Terminator/1  "countOut"
  In1/1 -> Multiply-Accumulate/2
  ? -> Terminator2/1  "vectorOutValid"

== system model_cnn/HDL CNN Model/Dense Layer 1/Dense Layer 1/adder117 ==
  In1 : Inport
  In2 : Inport  Port=2
  In3 : Inport  Port=3
  Data Type Conversion : DataTypeConversion  OutDataTypeStr=datatypeLayer3
  Multiply-Accumulate : hdlsllib/HDL Operations/Multiply-Accumulate  opMode=Streaming - using Number of Samples  initValueSetting=Dialog  initValue=0  initValueSetting2=Dialog  initValue2=0  initValueSetting3=Dialog  initValue3=0  num_samples=1984  RndMeth2=Floor  RndMeth3=Floor  datatype2=Inherit: Inherit via back propagation  datatype3=accumoutdatatype3  validOut=on  endInandOut=on  startOut=on  countOut=on  dim=-1  DoSatur=off  parallel=off
      settings: SourceProductBaseCode=SL
  Terminator : Terminator
  Terminator1 : Terminator
  Terminator2 : Terminator
  dataOut : Outport
  wires:
  Data Type Conversion/1 -> dataOut/1
  ? -> Terminator1/1  "validOut"
  In2/1 -> Multiply-Accumulate/1
  In3/1 -> ?
  Multiply-Accumulate/1 -> Data Type Conversion/1
  ? -> Terminator/1  "countOut"
  In1/1 -> Multiply-Accumulate/2
  ? -> Terminator2/1  "vectorOutValid"

== system model_cnn/HDL CNN Model/Dense Layer 1/Dense Layer 1/adder118 ==
  In1 : Inport
  In2 : Inport  Port=2
  In3 : Inport  Port=3
  Data Type Conversion : DataTypeConversion  OutDataTypeStr=datatypeLayer3
  Multiply-Accumulate : hdlsllib/HDL Operations/Multiply-Accumulate  opMode=Streaming - using Number of Samples  initValueSetting=Dialog  initValue=0  initValueSetting2=Dialog  initValue2=0  initValueSetting3=Dialog  initValue3=0  num_samples=1984  RndMeth2=Floor  RndMeth3=Floor  datatype2=Inherit: Inherit via back propagation  datatype3=accumoutdatatype3  validOut=on  endInandOut=on  startOut=on  countOut=on  dim=-1  DoSatur=off  parallel=off
      settings: SourceProductBaseCode=SL
  Terminator : Terminator
  Terminator1 : Terminator
  Terminator2 : Terminator
  dataOut : Outport
  wires:
  Data Type Conversion/1 -> dataOut/1
  ? -> Terminator1/1  "validOut"
  In2/1 -> Multiply-Accumulate/1
  In3/1 -> ?
  Multiply-Accumulate/1 -> Data Type Conversion/1
  ? -> Terminator/1  "countOut"
  In1/1 -> Multiply-Accumulate/2
  ? -> Terminator2/1  "vectorOutValid"

== system model_cnn/HDL CNN Model/Dense Layer 1/Dense Layer 1/adder119 ==
  In1 : Inport
  In2 : Inport  Port=2
  In3 : Inport  Port=3
  Data Type Conversion : DataTypeConversion  OutDataTypeStr=datatypeLayer3
  Multiply-Accumulate : hdlsllib/HDL Operations/Multiply-Accumulate  opMode=Streaming - using Number of Samples  initValueSetting=Dialog  initValue=0  initValueSetting2=Dialog  initValue2=0  initValueSetting3=Dialog  initValue3=0  num_samples=1984  RndMeth2=Floor  RndMeth3=Floor  datatype2=Inherit: Inherit via back propagation  datatype3=accumoutdatatype3  validOut=on  endInandOut=on  startOut=on  countOut=on  dim=-1  DoSatur=off  parallel=off
      settings: SourceProductBaseCode=SL
  Terminator : Terminator
  Terminator1 : Terminator
  Terminator2 : Terminator
  dataOut : Outport
  wires:
  Data Type Conversion/1 -> dataOut/1
  ? -> Terminator1/1  "validOut"
  In2/1 -> Multiply-Accumulate/1
  In3/1 -> ?
  Multiply-Accumulate/1 -> Data Type Conversion/1
  ? -> Terminator/1  "countOut"
  In1/1 -> Multiply-Accumulate/2
  ? -> Terminator2/1  "vectorOutValid"

== system model_cnn/HDL CNN Model/Dense Layer 1/Dense Layer 1/adder12 ==
  In1 : Inport
  In2 : Inport  Port=2
  In3 : Inport  Port=3
  Data Type Conversion : DataTypeConversion  OutDataTypeStr=datatypeLayer3
  Multiply-Accumulate : hdlsllib/HDL Operations/Multiply-Accumulate  opMode=Streaming - using Number of Samples  initValueSetting=Dialog  initValue=0  initValueSetting2=Dialog  initValue2=0  initValueSetting3=Dialog  initValue3=0  num_samples=1984  RndMeth2=Floor  RndMeth3=Floor  datatype2=Inherit: Inherit via back propagation  datatype3=accumoutdatatype3  validOut=on  endInandOut=on  startOut=on  countOut=on  dim=-1  DoSatur=off  parallel=off
      settings: SourceProductBaseCode=SL
  Terminator : Terminator
  Terminator1 : Terminator
  Terminator2 : Terminator
  dataOut : Outport
  wires:
  Data Type Conversion/1 -> dataOut/1
  ? -> Terminator1/1  "validOut"
  In2/1 -> Multiply-Accumulate/1
  In3/1 -> ?
  Multiply-Accumulate/1 -> Data Type Conversion/1
  ? -> Terminator/1  "countOut"
  In1/1 -> Multiply-Accumulate/2
  ? -> Terminator2/1  "vectorOutValid"

== system model_cnn/HDL CNN Model/Dense Layer 1/Dense Layer 1/adder120 ==
  In1 : Inport
  In2 : Inport  Port=2
  In3 : Inport  Port=3
  Data Type Conversion : DataTypeConversion  OutDataTypeStr=datatypeLayer3
  Multiply-Accumulate : hdlsllib/HDL Operations/Multiply-Accumulate  opMode=Streaming - using Number of Samples  initValueSetting=Dialog  initValue=0  initValueSetting2=Dialog  initValue2=0  initValueSetting3=Dialog  initValue3=0  num_samples=1984  RndMeth2=Floor  RndMeth3=Floor  datatype2=Inherit: Inherit via back propagation  datatype3=accumoutdatatype3  validOut=on  endInandOut=on  startOut=on  countOut=on  dim=-1  DoSatur=off  parallel=off
      settings: SourceProductBaseCode=SL
  Terminator : Terminator
  Terminator1 : Terminator
  Terminator2 : Terminator
  dataOut : Outport
  wires:
  Data Type Conversion/1 -> dataOut/1
  ? -> Terminator1/1  "validOut"
  In2/1 -> Multiply-Accumulate/1
  In3/1 -> ?
  Multiply-Accumulate/1 -> Data Type Conversion/1
  ? -> Terminator/1  "countOut"
  In1/1 -> Multiply-Accumulate/2
  ? -> Terminator2/1  "vectorOutValid"

== system model_cnn/HDL CNN Model/Dense Layer 1/Dense Layer 1/adder121 ==
  In1 : Inport
  In2 : Inport  Port=2
  In3 : Inport  Port=3
  Data Type Conversion : DataTypeConversion  OutDataTypeStr=datatypeLayer3
  Multiply-Accumulate : hdlsllib/HDL Operations/Multiply-Accumulate  opMode=Streaming - using Number of Samples  initValueSetting=Dialog  initValue=0  initValueSetting2=Dialog  initValue2=0  initValueSetting3=Dialog  initValue3=0  num_samples=1984  RndMeth2=Floor  RndMeth3=Floor  datatype2=Inherit: Inherit via back propagation  datatype3=accumoutdatatype3  validOut=on  endInandOut=on  startOut=on  countOut=on  dim=-1  DoSatur=off  parallel=off
      settings: SourceProductBaseCode=SL
  Terminator : Terminator
  Terminator1 : Terminator
  Terminator2 : Terminator
  dataOut : Outport
  wires:
  Data Type Conversion/1 -> dataOut/1
  ? -> Terminator1/1  "validOut"
  In2/1 -> Multiply-Accumulate/1
  In3/1 -> ?
  Multiply-Accumulate/1 -> Data Type Conversion/1
  ? -> Terminator/1  "countOut"
  In1/1 -> Multiply-Accumulate/2
  ? -> Terminator2/1  "vectorOutValid"

== system model_cnn/HDL CNN Model/Dense Layer 1/Dense Layer 1/adder122 ==
  In1 : Inport
  In2 : Inport  Port=2
  In3 : Inport  Port=3
  Data Type Conversion : DataTypeConversion  OutDataTypeStr=datatypeLayer3
  Multiply-Accumulate : hdlsllib/HDL Operations/Multiply-Accumulate  opMode=Streaming - using Number of Samples  initValueSetting=Dialog  initValue=0  initValueSetting2=Dialog  initValue2=0  initValueSetting3=Dialog  initValue3=0  num_samples=1984  RndMeth2=Floor  RndMeth3=Floor  datatype2=Inherit: Inherit via back propagation  datatype3=accumoutdatatype3  validOut=on  endInandOut=on  startOut=on  countOut=on  dim=-1  DoSatur=off  parallel=off
      settings: SourceProductBaseCode=SL
  Terminator : Terminator
  Terminator1 : Terminator
  Terminator2 : Terminator
  dataOut : Outport
  wires:
  Data Type Conversion/1 -> dataOut/1
  ? -> Terminator1/1  "validOut"
  In2/1 -> Multiply-Accumulate/1
  In3/1 -> ?
  Multiply-Accumulate/1 -> Data Type Conversion/1
  ? -> Terminator/1  "countOut"
  In1/1 -> Multiply-Accumulate/2
  ? -> Terminator2/1  "vectorOutValid"

== system model_cnn/HDL CNN Model/Dense Layer 1/Dense Layer 1/adder123 ==
  In1 : Inport
  In2 : Inport  Port=2
  In3 : Inport  Port=3
  Data Type Conversion : DataTypeConversion  OutDataTypeStr=datatypeLayer3
  Multiply-Accumulate : hdlsllib/HDL Operations/Multiply-Accumulate  opMode=Streaming - using Number of Samples  initValueSetting=Dialog  initValue=0  initValueSetting2=Dialog  initValue2=0  initValueSetting3=Dialog  initValue3=0  num_samples=1984  RndMeth2=Floor  RndMeth3=Floor  datatype2=Inherit: Inherit via back propagation  datatype3=accumoutdatatype3  validOut=on  endInandOut=on  startOut=on  countOut=on  dim=-1  DoSatur=off  parallel=off
      settings: SourceProductBaseCode=SL
  Terminator : Terminator
  Terminator1 : Terminator
  Terminator2 : Terminator
  dataOut : Outport
  wires:
  Data Type Conversion/1 -> dataOut/1
  ? -> Terminator1/1  "validOut"
  In2/1 -> Multiply-Accumulate/1
  In3/1 -> ?
  Multiply-Accumulate/1 -> Data Type Conversion/1
  ? -> Terminator/1  "countOut"
  In1/1 -> Multiply-Accumulate/2
  ? -> Terminator2/1  "vectorOutValid"

== system model_cnn/HDL CNN Model/Dense Layer 1/Dense Layer 1/adder124 ==
  In1 : Inport
  In2 : Inport  Port=2
  In3 : Inport  Port=3
  Data Type Conversion : DataTypeConversion  OutDataTypeStr=datatypeLayer3
  Multiply-Accumulate : hdlsllib/HDL Operations/Multiply-Accumulate  opMode=Streaming - using Number of Samples  initValueSetting=Dialog  initValue=0  initValueSetting2=Dialog  initValue2=0  initValueSetting3=Dialog  initValue3=0  num_samples=1984  RndMeth2=Floor  RndMeth3=Floor  datatype2=Inherit: Inherit via back propagation  datatype3=accumoutdatatype3  validOut=on  endInandOut=on  startOut=on  countOut=on  dim=-1  DoSatur=off  parallel=off
      settings: SourceProductBaseCode=SL
  Terminator : Terminator
  Terminator1 : Terminator
  Terminator2 : Terminator
  dataOut : Outport
  wires:
  Data Type Conversion/1 -> dataOut/1
  ? -> Terminator1/1  "validOut"
  In2/1 -> Multiply-Accumulate/1
  In3/1 -> ?
  Multiply-Accumulate/1 -> Data Type Conversion/1
  ? -> Terminator/1  "countOut"
  In1/1 -> Multiply-Accumulate/2
  ? -> Terminator2/1  "vectorOutValid"
